simulink model "Inverter_PWM_Generator"  (R2022b)
settings: Solver=VariableStepAuto  StartTime=0.0  StopTime=10.0  RelTol=1e-3
libraries: spsTriangleGeneratorLib x1
settings Model: Creator=Admin  LastModifiedBy=Admin

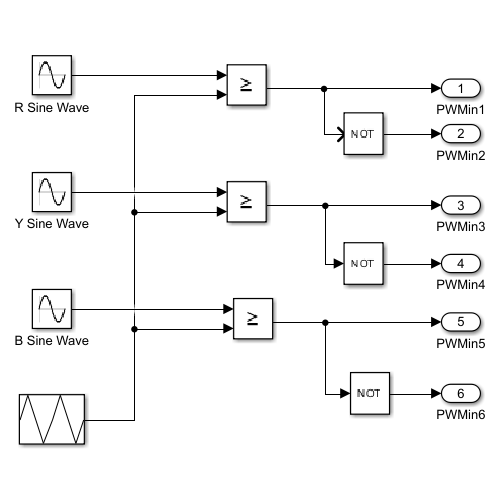
[thumbnail: Simulink's stored preview of the top-level diagram]
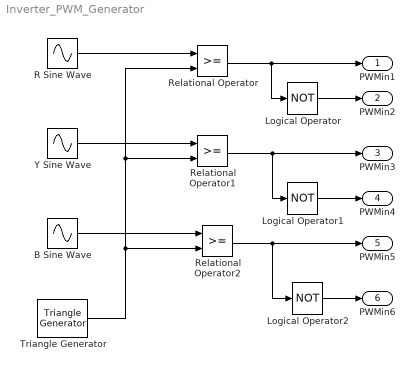
== system Inverter_PWM_Generator ==
  B Sine Wave : Sin  Amplitude=0.8  Frequency=2*pi*50  Phase=-2*pi*50/3  SampleTime=0
  Logical Operator : Logic  Operator=NOT  AllPortsSameDT=off  OutDataTypeStr=boolean
  Logical Operator1 : Logic  Operator=NOT  AllPortsSameDT=off  OutDataTypeStr=boolean
  Logical Operator2 : Logic  Operator=NOT  AllPortsSameDT=off  OutDataTypeStr=boolean
  R Sine Wave : Sin  Amplitude=0.8  Frequency=2*pi*50  SampleTime=0
  Relational Operator : RelationalOperator  OutDataTypeStr=boolean  RndMeth=Simplest  InputSameDT=off
  Relational Operator1 : RelationalOperator  OutDataTypeStr=boolean  RndMeth=Simplest  InputSameDT=off
  Relational Operator2 : RelationalOperator  OutDataTypeStr=boolean  RndMeth=Simplest  InputSameDT=off
  Triangle Generator : spsTriangleGeneratorLib/Triangle Generator  Freq=10e3  Phase=90  Ts=0
  Y Sine Wave : Sin  Amplitude=0.8  Frequency=2*pi*50  Phase=2*pi*50/3  SampleTime=0
  PWMin1 : Outport
  PWMin2 : Outport  Port=2
  PWMin3 : Outport  Port=3
  PWMin4 : Outport  Port=4
  PWMin5 : Outport  Port=5
  PWMin6 : Outport  Port=6
  wires:
  Logical Operator1/1 -> PWMin4/1
  Triangle Generator/1 -> Relational Operator2/2, Relational Operator1/2, Relational Operator/2
  Relational Operator1/1 -> PWMin3/1, Logical Operator1/1
  Logical Operator2/1 -> PWMin6/1
  R Sine Wave/1 -> Relational Operator/1
  Relational Operator/1 -> PWMin1/1, Logical Operator/1
  Relational Operator2/1 -> PWMin5/1, Logical Operator2/1
  Y Sine Wave/1 -> Relational Operator1/1
  B Sine Wave/1 -> Relational Operator2/1
  Logical Operator/1 -> PWMin2/1
